simulink model "DCMotorSpeedControl"  (Simulink 8.2)
settings: Solver=ode15s  StartTime=0.0  StopTime=10.0  RelTol=1e-3
values from neighbouring files (symbols this model uses):
  J = 52E-7    (= 5.2e-06)    [DesignDCMotorUsingPIDrlocusBode.m]    (also in DiscreteDesignandEquivalent.m; bode_mcode.m; il_zom_hae_byungsina.m; rlocus_mcode.m)
  Kd = Kd + 0.5    (= 0.512)    [DesignDCMotorUsingPIDrlocusBode.m]
  Ki = 2.5    [DesignDCMotorUsingPIDrlocusBode.m]
  Kp = 4    [DesignDCMotorUsingPIDrlocusBode.m]
  L = 10    [AEB_TTC_test.m]    (also in DesignDCMotorUsingPIDrlocusBode.m = 0.0024; DiscreteDesignandEquivalent.m = 0.0024; bode_mcode.m = 0.0024; errorvsstepsize.m = [H' D' E']')
  R = 1.8    [DesignDCMotorUsingPIDrlocusBode.m]    (also in DiscreteDesignandEquivalent.m; RCCircuit_data_plot2.m = 1; bode_mcode.m; il_zom_hae_byungsina.m)
undefined symbols (not defined in the file or in its folder): c, Kb, Kt
libraries: checkpacklib x1, simulink x1
settings Model: Creator=maen  LastModifiedBy=gyurse
settings DataIOCC: SignalLoggingSaveFormat=Dataset
settings ConfigurationSet: Description=SimMechanics 2G

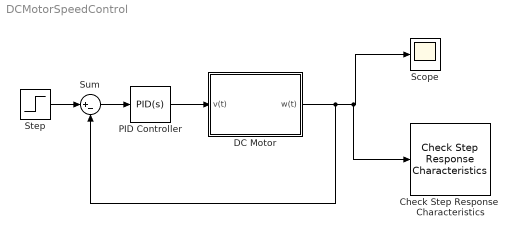
== system DCMotorSpeedControl ==
  Check Step Response  Characteristics : checkpacklib/Check Step Response  Characteristics  InstantiateOnLoad=on  enabled=on  stopWhenAssertionFail=off  export=off  ViewDlgPos=[172 392 510 390]  OpenViewOnLoad=off  LaunchViewOnOpen=off  TimeUnits=seconds  EnableStepResponseBound=on  InitialValue=0  FinalValue=1  StepTime=0  RiseTime=.7  PercentRise=90  SettlingTime=3.0  PercentSettling=2.0  PercentOvershoot=10  PercentUndershoot=0
  DC Motor : Subsystem
  PID Controller : simulink/Continuous/PID Controller  Controller=PID  TimeDomain=Continuous-time  SampleTime=1  IntegratorMethod=Forward Euler  FilterMethod=Forward Euler  Form=Parallel  P=Kp  I=Ki  D=Kd  N=100  InitialConditionSource=internal  InitialConditionForIntegrator=0  InitialConditionForFilter=0  ExternalReset=none  LimitOutput=off  UpperSaturationLimit=inf  LowerSaturationLimit=-inf  LinearizeAsGain=on  AntiWindupMode=none  Kb=1  TrackingMode=off  Kt=1  PParamMin=[]  PParamMax=[]  IParamMin=[]  IParamMax=[]  DParamMin=[]  DParamMax=[]  NParamMin=[]  NParamMax=[]  KbParamMin=[]  KbParamMax=[]  KtParamMin=[]  KtParamMax=[]  POutMin=[]  POutMax=[]  IOutMin=[]  IOutMax=[]  DOutMin=[]  DOutMax=[]  NOutMin=[]  NOutMax=[]  KbOutMin=[]  KbOutMax=[]  KtOutMin=[]  KtOutMax=[]  IntegratorOutMin=[]  IntegratorOutMax=[]  FilterOutMin=[]  FilterOutMax=[]  SumOutMin=[]  SumOutMax=[]  SumI1OutMin=[]  SumI1OutMax=[]  SumI2OutMin=[]  SumI2OutMax=[]  SumI3OutMin=[]  SumI3OutMax=[]  SumDOutMin=[]  SumDOutMax=[]  SaturationOutMin=[]  SaturationOutMax=[]  IntegratorContinuousStateAttributes=''  IntegratorStateMustResolveToSignalObject=off  IntegratorRTWStateStorageClass=Auto  FilterContinuousStateAttributes=''  FilterStateMustResolveToSignalObject=off  FilterRTWStateStorageClass=Auto
  Scope : Scope
  Step : Step  Time=0  SampleTime=0
  Sum : Sum  Inputs=|+-
  wires:
  Step/1 -> Sum/1
  Sum/1 -> PID Controller/1
  PID Controller/1 -> DC Motor/1(v(t))
  DC Motor/1(w(t)) -> Sum/2, Check Step Response  Characteristics/1, Scope/1

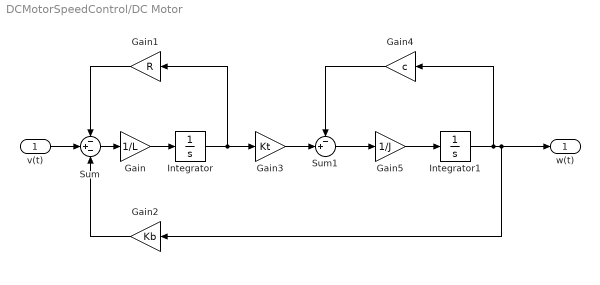
== system DCMotorSpeedControl/DC Motor ==
  v(t) : Inport
  Gain : Gain  Gain=1/L
  Gain1 : Gain  Gain=R
  Gain2 : Gain  Gain=Kb
  Gain3 : Gain  Gain=Kt
  Gain4 : Gain  Gain=c
  Gain5 : Gain  Gain=1/J
  Integrator : Integrator
  Integrator1 : Integrator
  Sum : Sum  Inputs=-+-
  Sum1 : Sum  Inputs=-+|
  w(t) : Outport
  wires:
  Gain4/1 -> Sum1/1
  Gain5/1 -> Integrator1/1
  Gain2/1 -> Sum/3
  Sum/1 -> Gain/1
  Gain3/1 -> Sum1/2
  Gain1/1 -> Sum/1
  Integrator1/1 -> Gain4/1, w(t)/1, Gain2/1
  Gain/1 -> Integrator/1
  Integrator/1 -> Gain1/1, Gain3/1
  Sum1/1 -> Gain5/1
  v(t)/1 -> Sum/2
